simulink model "novamontagemrobo"  (R2018a)
settings: Solver=VariableStepAuto  StartTime=0.0  StopTime=59  FixedStep=0.4  MaxStep=0.4  RelTol=1e-3
model workspace: external: MATLAB File C:\Users\reigo\Downloads\robotica2\simulink_CERTO\simulink\novamontagemrobo_DataFile.m (data not in the file)
undefined symbols (not defined in the file or in its folder): smiData, X, Y, Z
libraries: sm_lib x57, nesl_utility x31
(part 3 of 3)

== matlab function novamontagemrobo/MATLAB Function3 ==
  data: parametro_robo input; T output; mass_robo input; valor_q_inv input; dq input; ddq input; inercia_robo input
function T = T(parametro_robo,mass_robo,valor_q_inv,dq,ddq,inercia_robo)

%T(E1,E2,Itarefa,L2,L3,L4,ddq1,ddq2,ddq3,ddq4,ddq5,ddq6,dq1,dq2,dq3,dq4,dq5,dq6,m2,m3,m4,m5,m6,m7,mtarefa,q1,q2,q3,q4,q5,q6,xf,yf,zf)


% parametro_robo=[L1,L2,L3,L4,E1,E2,xf,yf,zf];
% mass_robo=[mass1 mass2 mass3 mass4 mass5 mass6 mass7 masstarefa];
% inercia_robo=[inercia1 inercia2 inercia3 inercia4 inercia5 inercia6 inercia7 inerciatarefa];

coder.extrinsic('evalin');
T1 = evalin('caller','T1');
T2 = evalin('caller','T2');
T3 = evalin('caller','T3');
T4 = evalin('caller','T4');
T5 = evalin('caller','T5');
T6 = evalin('caller','T6');




L1=parametro_robo(1);
L2=parametro_robo(2);
L3=parametro_robo(3);
L4=parametro_robo(4);
E1=parametro_robo(5);
E2=parametro_robo(6);
xf=parametro_robo(7);
yf=parametro_robo(8);
zf=parametro_robo(9);


q1=valor_q_inv(1);
q2=valor_q_inv(2);
q3=valor_q_inv(3);
q4=valor_q_inv(4);
q5=valor_q_inv(5);
q6=valor_q_inv(6);


dq1=dq(1);
dq2=dq(2);
dq3=dq(3);
dq4=dq(4);
dq5=dq(5);
dq6=dq(6);



ddq1=ddq(1);
ddq2=ddq(2);
ddq3=ddq(3);
ddq4=ddq(4);
ddq5=ddq(5);
ddq6=ddq(6);

m1=mass_robo(1);
m2=mass_robo(2);
m3=mass_robo(3);
m4=mass_robo(4);
m5=mass_robo(5);
m6=mass_robo(6);
m7=mass_robo(7);
mtarefa=mass_robo(8);


Itarefa=inercia_robo(22:24,:);
Itarefaxx=Itarefa(1,1);
Itarefaxy=Itarefa(1,2);
Itarefaxz=Itarefa(1,3);
Itarefayx=Itarefa(2,1);
Itarefayy=Itarefa(2,2);
Itarefayz=Itarefa(2,3);
Itarefazx=Itarefa(3,1);
Itarefazy=Itarefa(3,2);
Itarefazz=Itarefa(3,3);


T1 = T1(E1,E2,Itarefaxx,Itarefaxy,Itarefayx,Itarefaxz,Itarefayy,Itarefazx,Itarefayz,Itarefazy,Itarefazz,L2,L3,L4,ddq1,ddq2,ddq3,ddq4,ddq5,ddq6,dq1,dq2,dq3,dq4,dq5,dq6,m2,m3,m4,m5,m6,m7,mtarefa,q1,q2,q3,q4,q5,q6,xf,yf,zf);
%T2 = T2(Itarefa,ddq1,ddq2,ddq3,ddq4,ddq5,ddq6,dq1,dq2,dq3,dq4,dq5,dq6,mtarefa,q1,q2,q3,q4,q5,q6);
T2 = T2(E1,E2,Itarefaxx,Itarefaxy,Itarefayx,Itarefaxz,Itarefayy,Itarefazx,Itarefayz,Itarefazy,Itarefazz,L2,L3,L4,ddq1,ddq2,ddq3,ddq4,ddq5,ddq6,dq1,dq2,dq3,dq4,dq5,dq6,m2,m3,m4,m5,m6,m7,mtarefa,q1,q2,q3,q4,q5,q6,xf,yf,zf);
T3 = T3(E1,E2,Itarefaxx,Itarefaxy,Itarefayx,Itarefaxz,Itarefayy,Itarefazx,Itarefayz,Itarefazy,Itarefazz,L2,L3,L4,ddq1,ddq2,ddq3,ddq4,ddq5,ddq6,dq1,dq2,dq3,dq4,dq5,dq6,m3,m4,m5,m6,m7,mtarefa,q1,q2,q3,q4,q5,q6,xf,yf,zf);
T4 = T4(E1,E2,Itarefaxx,Itarefaxy,Itarefayx,Itarefaxz,Itarefayy,Itarefazx,Itarefayz,Itarefazy,Itarefazz,L2,L3,L4,ddq1,ddq2,ddq3,ddq4,ddq5,ddq6,dq1,dq2,dq3,dq4,dq5,dq6,m4,m5,m6,m7,mtarefa,q1,q2,q3,q4,q5,q6,xf,yf,zf);
T5 = T5(E1,E2,Itarefaxx,Itarefaxy,Itarefayx,Itarefaxz,Itarefayy,Itarefazx,Itarefayz,Itarefazy,Itarefazz,L2,L3,L4,ddq1,ddq2,ddq3,ddq4,ddq5,ddq6,dq1,dq2,dq3,dq4,dq5,dq6,m5,m6,m7,mtarefa,q1,q2,q3,q4,q5,q6,xf,yf,zf);
T6 = T6(E1,E2,Itarefaxx,Itarefaxy,Itarefayx,Itarefaxz,Itarefayy,Itarefazx,Itarefayz,Itarefazy,Itarefazz,L2,L3,L4,ddq1,ddq2,ddq3,ddq4,ddq5,ddq6,dq1,dq2,dq3,dq4,dq5,dq6,m6,m7,mtarefa,q1,q2,q3,q4,q5,q6,xf,yf,zf);

T=zeros(6,1);
T = [T1; T2; T3; T4; T5; T6];

== matlab function novamontagemrobo/MATLAB Function4 ==
  data: matriz input; dq output; velocidades input
function dq = fcn(matriz,velocidades)

dq=matriz\velocidades';

== matlab function novamontagemrobo/MATLAB Function6 ==
  data: matriz input; ddq output; dq input; dmatriz input; aceleracao input
function ddq = acel_juntas(matriz,dq,dmatriz,aceleracao)


ddq=matriz\aceleracao'-matriz\dmatriz*dq;

== matlab function novamontagemrobo/djacob ==
  data: parametro_robo input; dJtot output; valor_q_inv input; dq input
function dJtot = djacob(parametro_robo,valor_q_inv,dq)
%#codegen

%    This function was generated by the Symbolic Math Toolbox version 8.1.
%    12-Jan-2021 01:39:36


L1=parametro_robo(1);
L2=parametro_robo(2);
L3=parametro_robo(3);
L4=parametro_robo(4);
E1=parametro_robo(5);
E2=parametro_robo(6);
xf=parametro_robo(7);
yf=parametro_robo(8);
zf=parametro_robo(9);


q1=valor_q_inv(1);
q2=valor_q_inv(2);
q3=valor_q_inv(3);
q4=valor_q_inv(4);
q5=valor_q_inv(5);
q6=valor_q_inv(6);


dq1=dq(1);
dq2=dq(2);
dq3=dq(3);
dq4=dq(4);
dq5=dq(5);
dq6=dq(6);




t2 = q2+q3;
t3 = sin(q1);
t4 = sin(q5);
t5 = cos(q1);
t6 = sin(q4);
t7 = t5.*t6;
t8 = sin(t2);
t9 = cos(q4);
t13 = t3.*t8.*t9;
t10 = t7-t13;
t11 = cos(t2);
t12 = cos(q5);
t14 = t4.*t10;
t15 = t3.*t11.*t12;
t16 = t14+t15;
t17 = sin(q6);
t18 = cos(q6);
t19 = t10.*t12;
t24 = t3.*t4.*t11;
t20 = t19-t24;
t21 = t5.*t9;
t22 = t3.*t6.*t8;
t23 = t21+t22;
t25 = L4+xf;
t26 = t3.*t4.*t8;
t42 = t3.*t9.*t11.*t12;
t27 = t26-t42;
t28 = cos(q2);
t29 = sin(q2);
t30 = t3.*t6;
t31 = t5.*t8.*t9;
t32 = t30+t31;
t33 = t3.*t9;
t102 = t5.*t6.*t8;
t34 = t33-t102;
t35 = t12.*t32;
t36 = t4.*t5.*t11;
t37 = t35+t36;
t38 = t3.*t8.*t12;
t39 = t3.*t4.*t9.*t11;
t40 = t38+t39;
t41 = t25.*t40;
t43 = t17.*t27;
t59 = t3.*t6.*t11.*t18;
t44 = t43-t59;
t45 = t44.*yf;
t46 = t18.*t27;
t47 = t3.*t6.*t11.*t17;
t48 = t46+t47;
t49 = t48.*zf;
t50 = t5.*t8.*t9.*t12;
t51 = t36+t50;
t52 = t5.*t8.*t12;
t53 = t4.*t5.*t9.*t11;
t54 = t52+t53;
t55 = L3.*t8;
t56 = L2.*t29;
t154 = E2.*t28;
t57 = t55+t56-t154;
t58 = t3.*t57;
t60 = t41+t45+t49+t58;
t61 = t4.*t5.*t8;
t63 = t5.*t9.*t11.*t12;
t62 = t61-t63;
t64 = t5.*t11.*t12;
t77 = t4.*t5.*t8.*t9;
t65 = t64-t77;
t66 = t25.*t65;
t67 = t17.*t51;
t68 = t5.*t6.*t8.*t18;
t69 = t67+t68;
t70 = t69.*yf;
t71 = t18.*t51;
t78 = t5.*t6.*t8.*t17;
t72 = t71-t78;
t73 = t72.*zf;
t74 = L3.*t11;
t75 = L2.*t28;
t76 = E2.*t29;
t79 = L3.*t5.*t11;
t80 = t66+t70+t73+t79;
t81 = t18.*t54.*zf;
t82 = t17.*t54.*yf;
t119 = t25.*t62;
t83 = t81+t82-t119;
t84 = t5.*t9.*t11.*t18;
t103 = t5.*t6.*t11.*t12.*t17;
t85 = t84-t103;
t86 = t85.*yf;
t87 = t5.*t9.*t11.*t17;
t88 = t5.*t6.*t11.*t12.*t18;
t89 = t87+t88;
t90 = t4.*t5.*t6.*t11.*t25;
t104 = t89.*zf;
t91 = t86+t90-t104;
t92 = dq4.*t91;
t93 = L3.*t3.*t8;
t94 = t41+t45+t49+t93;
t95 = t18.*t62;
t96 = t5.*t6.*t11.*t17;
t97 = t95+t96;
t98 = t97.*yf;
t99 = t17.*t62;
t145 = t5.*t6.*t11.*t18;
t100 = t99-t145;
t146 = t100.*zf;
t101 = t98-t146;
t105 = t10.*t18;
t106 = t12.*t17.*t23;
t107 = t105+t106;
t108 = t10.*t17;
t190 = t12.*t18.*t23;
t109 = t108-t190;
t110 = t109.*zf;
t111 = t4.*t23.*t25;
t112 = t110+t111-t107.*yf;
t113 = t18.*t34;
t114 = t17.*t34;
t115 = t20.*t25;
t116 = t16.*t18.*zf;
t117 = t16.*t17.*yf;
t118 = t115+t116+t117;
t120 = t12.*t25.*t34;
t121 = t4.*t18.*t34.*zf;
t122 = t4.*t17.*t34.*yf;
t123 = t120+t121+t122;
t124 = t4.*t32;
t125 = t64-t124;
t148 = t17.*t37;
t126 = t113-t148;
t127 = t126.*yf;
t128 = t18.*t37;
t129 = t114+t128;
t130 = t17.*t32;
t155 = t12.*t18.*t34;
t131 = t130-t155;
t132 = t131.*yf;
t133 = t18.*t32;
t134 = t12.*t17.*t34;
t135 = t133+t134;
t136 = t135.*zf;
t137 = t132+t136;
t138 = t17.*t23;
t139 = t18.*t20;
t140 = t138+t139;
t141 = t140.*yf;
t142 = t17.*t20;
t150 = t18.*t23;
t143 = t142-t150;
t144 = t141-t143.*zf;
t147 = t18.*t125.*yf;
t149 = E1+t74+t75+t76;
t151 = t25.*t54;
t152 = t100.*yf;
t153 = t97.*zf;
t156 = t74+t75+t76;
t157 = t3.*t8.*t9.*t12;
t158 = t24+t157;
t184 = t3.*t4.*t8.*t9;
t159 = t15-t184;
t160 = t25.*t159;
t161 = t17.*t158;
t162 = t3.*t6.*t8.*t18;
t163 = t161+t162;
t164 = t163.*yf;
t165 = t18.*t158;
t185 = t3.*t6.*t8.*t17;
t166 = t165-t185;
t167 = t166.*zf;
t168 = t5.*t57;
t169 = t151+t152+t153+t168;
t170 = L3.*t5.*t8;
t171 = t151+t152+t153+t170;
t172 = t18.*t40.*zf;
t173 = t17.*t40.*yf;
t197 = t25.*t27;
t174 = t172+t173-t197;
t175 = t3.*t9.*t11.*t18;
t191 = t3.*t6.*t11.*t12.*t17;
t176 = t175-t191;
t177 = t176.*yf;
t178 = t3.*t9.*t11.*t17;
t179 = t3.*t6.*t11.*t12.*t18;
t180 = t178+t179;
t181 = t3.*t4.*t6.*t11.*t25;
t192 = t180.*zf;
t182 = t177+t181-t192;
t183 = dq4.*t182;
t186 = L3.*t3.*t11;
t187 = t160+t164+t167+t186;
t188 = t48.*yf;
t212 = t44.*zf;
t189 = t188-t212;
t193 = t131.*zf;
t194 = t4.*t25.*t34;
t195 = t193+t194-t135.*yf;
t196 = t16.*t25;
t198 = t12.*t23.*t25;
t199 = t4.*t18.*t23.*zf;
t200 = t4.*t17.*t23.*yf;
t201 = t198+t199+t200;
t202 = t18.*t125.*zf;
t203 = t17.*t125.*yf;
t204 = t129.*yf;
t205 = t126.*zf;
t206 = t204+t205;
t207 = t109.*yf;
t208 = t107.*zf;
t209 = t207+t208;
t210 = t16.*t18.*yf;
t211 = t210-t16.*t17.*zf;
t213 = t11.*t12;
t232 = t4.*t8.*t9;
t214 = t213-t232;
t215 = t4.*t8;
t217 = t9.*t11.*t12;
t216 = t215-t217;
t218 = t17.*t216;
t244 = t6.*t11.*t18;
t219 = t218-t244;
t220 = t219.*yf;
t221 = t18.*t216;
t222 = t6.*t11.*t17;
t223 = t221+t222;
t224 = t223.*zf;
t225 = t8.*t12;
t226 = t4.*t9.*t11;
t227 = t225+t226;
t228 = t25.*t227;
t229 = t4.*t11;
t230 = t8.*t9.*t12;
t231 = t229+t230;
t233 = t18.*t214.*zf;
t234 = t17.*t214.*yf;
t255 = t25.*t231;
t235 = t233+t234-t255;
t236 = t8.*t9.*t18;
t253 = t6.*t8.*t12.*t17;
t237 = t236-t253;
t238 = t237.*yf;
t239 = t8.*t9.*t17;
t240 = t6.*t8.*t12.*t18;
t241 = t239+t240;
t242 = t4.*t6.*t8.*t25;
t254 = t241.*zf;
t243 = t238+t242-t254;
t245 = t55+t220+t224+t228;
t246 = dq3.*t245;
t247 = t18.*t231;
t270 = t6.*t8.*t17;
t248 = t247-t270;
t249 = t17.*t231;
t250 = t6.*t8.*t18;
t251 = t249+t250;
t271 = t248.*yf;
t272 = t251.*zf;
t252 = t271-t272;
t256 = t6.*t11.*t12.*t25;
t257 = t4.*t6.*t11.*t18.*zf;
t258 = t4.*t6.*t11.*t17.*yf;
t259 = t256+t257+t258;
t260 = t9.*t11.*t17;
t261 = t6.*t11.*t12.*t18;
t262 = t260+t261;
t263 = t262.*yf;
t264 = t9.*t11.*t18;
t265 = t264-t6.*t11.*t12.*t17;
t266 = t265.*zf;
t267 = t263+t266;
t268 = t18.*t227.*yf;
t269 = t268-t17.*t227.*zf;
dJtot = reshape([dq2.*t60+dq3.*t94-dq4.*t112-dq5.*t118+dq6.*t144+dq1.*(t127-t5.*t149-t129.*zf+t25.*(t124-t5.*t11.*t12)),-dq2.*t169-dq3.*t171-dq4.*t195+dq6.*t206+dq5.*(t202+t203-t25.*t37)-dq1.*(t196+t3.*t149-t143.*yf-t140.*zf),0.0,0.0,0.0,0.0,t92+dq1.*t60-dq3.*t80-dq5.*t83-dq6.*t101-dq2.*(t66+t70+t73+t5.*t156),t183-dq1.*t169-dq5.*t174-dq3.*t187-dq6.*t189-dq2.*(t160+t164+t167+t3.*t156),t246-dq5.*t235-dq4.*t243-dq6.*t252+dq2.*(t55+t56-t154+t220+t224+t228),-dq1.*t5,-dq1.*t3,0.0,t92-dq2.*t80-dq3.*t80-dq5.*t83+dq1.*t94-dq6.*t101,t183-dq1.*t171-dq5.*t174-dq2.*t187-dq3.*t187-dq6.*t189,t246-dq5.*t235+dq2.*t245-dq4.*t243-dq6.*t252,-dq1.*t5,-dq1.*t3,0.0,dq2.*t91+dq3.*t91-dq1.*t112-dq5.*t123-dq6.*t137+dq4.*(yf.*(t113-t12.*t17.*t32)-zf.*(t114+t12.*t18.*t32)+t4.*t25.*t32),dq2.*t182+dq3.*t182-dq1.*t195+dq5.*t201+dq6.*t209-dq4.*(yf.*(t150-t10.*t12.*t17)-zf.*(t138+t10.*t12.*t18)+t4.*t10.*t25),dq4.*(-yf.*(t244+t9.*t11.*t12.*t17)+zf.*(t222-t9.*t11.*t12.*t18)+t4.*t9.*t11.*t25)-dq2.*t243-dq3.*t243+dq5.*t259-dq6.*t267,-dq1.*t3.*t11-dq2.*t5.*t8-dq3.*t5.*t8,-dq2.*t3.*t8-dq3.*t3.*t8+dq1.*t5.*t11,-dq2.*t11-dq3.*t11,-dq2.*t83-dq3.*t83-dq1.*t118-dq4.*t123+dq6.*(t147-t17.*t125.*zf)-dq5.*(t25.*t125+t17.*t37.*yf+t18.*t37.*zf),-dq2.*t174-dq3.*t174+dq4.*t201+dq6.*t211+dq1.*(t202+t203-t25.*t37)+dq5.*(-t196+t17.*t20.*yf+t18.*t20.*zf),dq5.*(t228+t17.*t216.*yf+t18.*t216.*zf)-dq2.*t235-dq3.*t235+dq4.*t259-dq6.*t269,-dq1.*t23+dq4.*t32+dq2.*t5.*t6.*t11+dq3.*t5.*t6.*t11,-dq4.*t10-dq1.*t34+dq2.*t3.*t6.*t11+dq3.*t3.*t6.*t11,-dq2.*t6.*t8-dq3.*t6.*t8+dq4.*t9.*t11,-dq2.*t101-dq3.*t101-dq4.*t137+dq1.*t144+dq5.*(t147-t17.*zf.*(t64-t124))+dq6.*(t127-t129.*zf),-dq2.*t189-dq3.*t189+dq1.*t206+dq4.*t209+dq5.*t211+dq6.*(t143.*yf+t140.*zf),dq6.*(t220+t224)-dq2.*t252-dq3.*t252-dq4.*t267-dq5.*t269,-dq1.*t16-dq5.*t37-dq2.*t54-dq3.*t54-dq4.*t4.*t34,dq5.*t20-dq2.*t40-dq3.*t40+dq1.*(t64-t124)+dq4.*t4.*t23,-dq2.*t214-dq3.*t214+dq5.*t216+dq4.*t4.*t6.*t11],[6,6]);

== matlab function novamontagemrobo/jacob ==
  data: parametro_robo input; Jtot output; valor_q_inv input
function Jtot = jacob(parametro_robo,valor_q_inv)
%#codegen

%    This function was generated by the Symbolic Math Toolbox version 8.1.
%    12-Jan-2021 01:39:21


L1=parametro_robo(1);
L2=parametro_robo(2);
L3=parametro_robo(3);
L4=parametro_robo(4);
E1=parametro_robo(5);
E2=parametro_robo(6);
xf=parametro_robo(7);
yf=parametro_robo(8);
zf=parametro_robo(9);


q1=valor_q_inv(1);
q2=valor_q_inv(2);
q3=valor_q_inv(3);
q4=valor_q_inv(4);
q5=valor_q_inv(5);
q6=valor_q_inv(6);



t2 = q2+q3;
t3 = sin(q1);
t4 = cos(t2);
t5 = cos(q1);
t6 = cos(q4);
t7 = sin(t2);
t8 = sin(q4);
t9 = cos(q5);
t10 = t5.*t8;
t18 = t3.*t6.*t7;
t11 = t10-t18;
t12 = sin(q5);
t13 = sin(q6);
t14 = t5.*t6;
t15 = t3.*t7.*t8;
t16 = t14+t15;
t17 = cos(q6);
t19 = t9.*t11;
t70 = t3.*t4.*t12;
t20 = t19-t70;
t21 = L4+xf;
t22 = t5.*t7.*t12;
t29 = t4.*t5.*t6.*t9;
t23 = t22-t29;
t24 = cos(q2);
t25 = sin(q2);
t26 = t5.*t7.*t9;
t27 = t4.*t5.*t6.*t12;
t28 = t26+t27;
t30 = t13.*t23;
t31 = t30-t4.*t5.*t8.*t17;
t32 = t17.*t23;
t33 = t4.*t5.*t8.*t13;
t34 = t32+t33;
t35 = t3.*t8;
t36 = t5.*t6.*t7;
t37 = t35+t36;
t38 = t3.*t6;
t40 = t5.*t7.*t8;
t39 = t38-t40;
t41 = t12.*t37;
t46 = t4.*t5.*t9;
t42 = t41-t46;
t43 = t9.*t37;
t44 = t4.*t5.*t12;
t45 = t43+t44;
t47 = L3.*t4;
t48 = L2.*t24;
t49 = E2.*t25;
t50 = E1+t47+t48+t49;
t51 = t17.*t39;
t52 = t51-t13.*t45;
t53 = t13.*t39;
t54 = t17.*t45;
t55 = t53+t54;
t56 = L3.*t7;
t57 = L2.*t25;
t58 = t56+t57-E2.*t24;
t59 = t3.*t7.*t12;
t64 = t3.*t4.*t6.*t9;
t60 = t59-t64;
t61 = t3.*t7.*t9;
t62 = t3.*t4.*t6.*t12;
t63 = t61+t62;
t65 = t13.*t60;
t66 = t65-t3.*t4.*t8.*t17;
t67 = t17.*t60;
t68 = t3.*t4.*t8.*t13;
t69 = t67+t68;
t71 = t11.*t12;
t72 = t3.*t4.*t9;
t73 = t71+t72;
t74 = t13.*t16;
t75 = t17.*t20;
t76 = t74+t75;
t77 = t13.*t20;
t78 = t4.*t12;
t79 = t6.*t7.*t9;
t80 = t78+t79;
t81 = t13.*t80;
t82 = t7.*t8.*t17;
t83 = t81+t82;
t84 = t17.*t80;
t85 = t84-t7.*t8.*t13;
t86 = t4.*t9;
t87 = t86-t6.*t7.*t12;
t88 = t7.*t9;
t89 = t4.*t6.*t12;
t90 = t88+t89;
t91 = t7.*t12;
t93 = t4.*t6.*t9;
t92 = t91-t93;
Jtot = reshape([-t3.*t50-t21.*t73+t76.*zf+yf.*(t77-t16.*t17),t5.*t50-t21.*t42-t52.*yf+t55.*zf,0.0,0.0,0.0,1.0,-t21.*t28-t5.*t58-t31.*yf-t34.*zf,-t3.*t58-t21.*t63-t66.*yf-t69.*zf,-t47-t48-t49-t21.*t87-t83.*yf-t85.*zf,-t3,t5,0.0,-t21.*t28-t31.*yf-t34.*zf-L3.*t5.*t7,-t21.*t63-t66.*yf-t69.*zf-L3.*t3.*t7,-t47-t21.*t87-t83.*yf-t85.*zf,-t3,t5,0.0,yf.*(t17.*t37+t9.*t13.*t39)-zf.*(t13.*t37-t9.*t17.*t39)-t12.*t21.*t39,-yf.*(t11.*t17+t9.*t13.*t16)+zf.*(t11.*t13-t9.*t16.*t17)+t12.*t16.*t21,yf.*(t4.*t6.*t17-t4.*t8.*t9.*t13)-zf.*(t4.*t6.*t13+t4.*t8.*t9.*t17)+t4.*t8.*t12.*t21,t4.*t5,t3.*t4,-t7,-t21.*t45-t13.*t42.*yf-t17.*t42.*zf,t20.*t21+t13.*t73.*yf+t17.*t73.*zf,t21.*t92-t13.*t90.*yf-t17.*t90.*zf,-t38+t40,t16,t4.*t8,t55.*yf+t52.*zf,-t76.*yf+zf.*(t77-t16.*t17),-yf.*(t17.*t92+t4.*t8.*t13)+zf.*(t13.*t92-t4.*t8.*t17),-t41+t46,t73,-t88-t89],[6,6]);

== matlab function novamontagemrobo/MATLAB Function7 ==
  data: parametro_robo output; config_tarefa output; massa_robo output; inercia_robo output
function [parametro_robo,config_tarefa,massa_robo,inercia_robo] = condicao_inicial
L1=0.590; L2=1.350; L3=1.600;L4=0.215;
E1=0.750; E2=-0.041;
xf=0.22485;yf=0;zf=0;


mass1=207.61613;
mass2=346.81729;
mass3=366.65763;
mass4=243.34094;
mass5=10.76884;
mass6=27.61521;
mass7=3.40236; %flange+ferramenta
masstarefa=8.90300;
%masstarefa=0;



inercia1=[6.45927 0.00073 -0.42267; 0.00073 8.55120 0.00155; -0.42267 0.00155 13.15421];

%

inercia2=[11.08697 3.39167 5.38787; 3.39167 37.87049 0.88684; 5.38787 0.88684 35.38487];  % Kg*m^2 
inercia3=[6.70839 -7.30351 -0.12339; -7.30351 78.03742 0.03995; -0.12339 0.03995 78.85343];
inercia4=[2.40106 1.64045 -1.15010; 1.64045 48.35669 -0.11971; -1.15010 -0.11971 47.88720];
inercia5=[0.02668 0.00251 0.00000; 0.00251 0.11156 0.00000; 0.00000 0.00000 0.10998];
inercia6=[0.26923 -0.04332 -0.00012; -0.04332 0.22283 -0.00011; -0.00012 -0.00011 0.37601];
inercia7=[0.05118 -0.0005 -0.00002; -0.00005 0.01547 0.00003; -0.00002 0.00003 0.06098]; %flange+ferramenta
inerciatarefa=[0.22649 -0.00006 -0.00005;-0.00006 0.17109 -0.00013;-0.00005 -0.00013 0.23614];

%inerciatarefa=zeros(3,3);








%ligar desligar mtarefa e inerciatarefa daqui. alterar função para receber
%tempo


parametro_robo=[L1,L2,L3,L4,E1,E2,xf,yf,zf];
massa_robo=[mass1 mass2 mass3 mass4 mass5 mass6 mass7 masstarefa];
inercia_robo=[inercia1; inercia2 ;inercia3 ;inercia4 ;inercia5 ;inercia6 ;inercia7 ;inerciatarefa];
%inercia_robo=inerciatarefa;
xC = 0; yC = 0; zC = 0; qxC = 0; qyC = 0; qzC = 0; 
alt_min_eixo2=0.585;
config_tarefa=[xC,yC,zC,qxC,qyC,qzC,alt_min_eixo2];

end

== matlab function novamontagemrobo/MATLAB Function9 ==
  data: parametro_robo input; G output; mass_robo input; valor_q_inv input
function G = G(parametro_robo,mass_robo,valor_q_inv)

coder.extrinsic('evalin');
G1 = evalin('caller','G1'); 
G2 = evalin('caller','G2');
G3 = evalin('caller','G3');
G4 = evalin('caller','G4');
G5 = evalin('caller','G5');
G6 = evalin('caller','G6');




L1=parametro_robo(1);
L2=parametro_robo(2);
L3=parametro_robo(3);
L4=parametro_robo(4);
E1=parametro_robo(5);
E2=parametro_robo(6);
xf=parametro_robo(7);
yf=parametro_robo(8);
zf=parametro_robo(9);


q1=valor_q_inv(1);
q2=valor_q_inv(2);
q3=valor_q_inv(3);
q4=valor_q_inv(4);
q5=valor_q_inv(5);
q6=valor_q_inv(6);



m1=mass_robo(1);
m2=mass_robo(2);
m3=mass_robo(3);
m4=mass_robo(4);
m5=mass_robo(5);
m6=mass_robo(6);
m7=mass_robo(7);
mtarefa=mass_robo(8);




G1 = G1();
G2 = G2(E2,L2,L3,L4,m2,m3,m4,m5,m6,m7,mtarefa,q2,q3,q4,q5,q6,xf,yf,zf);
G3 = G3(E2,L3,L4,m3,m4,m5,m6,m7,mtarefa,q2,q3,q4,q5,q6,xf,yf,zf);
G4 = G4(L4,m4,m5,m6,m7,mtarefa,q2,q3,q4,q5,q6,xf,yf,zf);
G5 = G5(L4,m5,m6,m7,mtarefa,q2,q3,q4,q5,q6,xf,yf,zf);
G6 = G6(m6,m7,mtarefa,q2,q3,q4,q5,q6,yf,zf);

G=zeros(6,1);
G = [G1; G2; G3; G4; G5; G6];

== matlab function novamontagemrobo/MATLAB Function10 ==
  data: T input; H output; M input; ddq input; G input
function H = H(T, M ,ddq, G)

H = T-M*ddqm-G;

== matlab function novamontagemrobo/MATLAB Function11 ==
  data: T input; H output; M input; ddq input; G input
function H = H(T, M ,ddq, G)

H = T-M*ddq-G;

== matlab function novamontagemrobo/MATLAB Function12 ==
  data: parametro_robo input; T output; mass_robo input; qm input; dqm input; ddqm input; inercia_robo input
function T = T(parametro_robo,mass_robo,qm,dqm,ddqm,inercia_robo)

%T(E1,E2,Itarefa,L2,L3,L4,ddq1,ddq2,ddq3,ddq4,ddq5,ddq6,dq1,dq2,dq3,dq4,dq5,dq6,m2,m3,m4,m5,m6,m7,mtarefa,q1,q2,q3,q4,q5,q6,xf,yf,zf)


% parametro_robo=[L1,L2,L3,L4,E1,E2,xf,yf,zf];
% mass_robo=[mass1 mass2 mass3 mass4 mass5 mass6 mass7 masstarefa];
% inercia_robo=[inercia1 inercia2 inercia3 inercia4 inercia5 inercia6 inercia7 inerciatarefa];


coder.extrinsic('evalin');
T1 = evalin('caller','T1');
T2 = evalin('caller','T2');
T3 = evalin('caller','T3');
T4 = evalin('caller','T4');
T5 = evalin('caller','T5');
T6 = evalin('caller','T6');



L1=parametro_robo(1);
L2=parametro_robo(2);
L3=parametro_robo(3);
L4=parametro_robo(4);
E1=parametro_robo(5);
E2=parametro_robo(6);
xf=parametro_robo(7);
yf=parametro_robo(8);
zf=parametro_robo(9);


q1=qm(1);
q2=qm(2);
q3=qm(3);
q4=qm(4);
q5=qm(5);
q6=qm(6);


dq1=dqm(1);
dq2=dqm(2);
dq3=dqm(3);
dq4=dqm(4);
dq5=dqm(5);
dq6=dqm(6);



ddq1=ddqm(1);
ddq2=ddqm(2);
ddq3=ddqm(3);
ddq4=ddqm(4);
ddq5=ddqm(5);
ddq6=ddqm(6);

m1=mass_robo(1);
m2=mass_robo(2);
m3=mass_robo(3);
m4=mass_robo(4);
m5=mass_robo(5);
m6=mass_robo(6);
m7=mass_robo(7);
mtarefa=mass_robo(8);


Itarefa=inercia_robo(22:24,:);
Itarefaxx=Itarefa(1,1);
Itarefaxy=Itarefa(1,2);
Itarefaxz=Itarefa(1,3);
Itarefayx=Itarefa(2,1);
Itarefayy=Itarefa(2,2);
Itarefayz=Itarefa(2,3);
Itarefazx=Itarefa(3,1);
Itarefazy=Itarefa(3,2);
Itarefazz=Itarefa(3,3);


T1 = T1(E1,E2,Itarefaxx,Itarefaxy,Itarefayx,Itarefaxz,Itarefayy,Itarefazx,Itarefayz,Itarefazy,Itarefazz,L2,L3,L4,ddq1,ddq2,ddq3,ddq4,ddq5,ddq6,dq1,dq2,dq3,dq4,dq5,dq6,m2,m3,m4,m5,m6,m7,mtarefa,q1,q2,q3,q4,q5,q6,xf,yf,zf);
%T2 = T2(Itarefa,ddq1,ddq2,ddq3,ddq4,ddq5,ddq6,dq1,dq2,dq3,dq4,dq5,dq6,mtarefa,q1,q2,q3,q4,q5,q6);
T2 = T2(E1,E2,Itarefaxx,Itarefaxy,Itarefayx,Itarefaxz,Itarefayy,Itarefazx,Itarefayz,Itarefazy,Itarefazz,L2,L3,L4,ddq1,ddq2,ddq3,ddq4,ddq5,ddq6,dq1,dq2,dq3,dq4,dq5,dq6,m2,m3,m4,m5,m6,m7,mtarefa,q1,q2,q3,q4,q5,q6,xf,yf,zf);
T3 = T3(E1,E2,Itarefaxx,Itarefaxy,Itarefayx,Itarefaxz,Itarefayy,Itarefazx,Itarefayz,Itarefazy,Itarefazz,L2,L3,L4,ddq1,ddq2,ddq3,ddq4,ddq5,ddq6,dq1,dq2,dq3,dq4,dq5,dq6,m3,m4,m5,m6,m7,mtarefa,q1,q2,q3,q4,q5,q6,xf,yf,zf);
T4 = T4(E1,E2,Itarefaxx,Itarefaxy,Itarefayx,Itarefaxz,Itarefayy,Itarefazx,Itarefayz,Itarefazy,Itarefazz,L2,L3,L4,ddq1,ddq2,ddq3,ddq4,ddq5,ddq6,dq1,dq2,dq3,dq4,dq5,dq6,m4,m5,m6,m7,mtarefa,q1,q2,q3,q4,q5,q6,xf,yf,zf);
T5 = T5(E1,E2,Itarefaxx,Itarefaxy,Itarefayx,Itarefaxz,Itarefayy,Itarefazx,Itarefayz,Itarefazy,Itarefazz,L2,L3,L4,ddq1,ddq2,ddq3,ddq4,ddq5,ddq6,dq1,dq2,dq3,dq4,dq5,dq6,m5,m6,m7,mtarefa,q1,q2,q3,q4,q5,q6,xf,yf,zf);
T6 = T6(E1,E2,Itarefaxx,Itarefaxy,Itarefayx,Itarefaxz,Itarefayy,Itarefazx,Itarefayz,Itarefazy,Itarefazz,L2,L3,L4,ddq1,ddq2,ddq3,ddq4,ddq5,ddq6,dq1,dq2,dq3,dq4,dq5,dq6,m6,m7,mtarefa,q1,q2,q3,q4,q5,q6,xf,yf,zf);

T=zeros(6,1);
T = [T1; T2; T3; T4; T5; T6];

== matlab function novamontagemrobo/MATLAB Function13 ==
  data: parametro_robo input; M output; mass_robo input; qm input; inercia_robo input
function M = M(parametro_robo,mass_robo,qm,inercia_robo)

%T(E1,E2,Itarefa,L2,L3,L4,ddq1,ddq2,ddq3,ddq4,ddq5,ddq6,dq1,dq2,dq3,dq4,dq5,dq6,m2,m3,m4,m5,m6,m7,mtarefa,q1,q2,q3,q4,q5,q6,xf,yf,zf)


% parametro_robo=[L1,L2,L3,L4,E1,E2,xf,yf,zf];
% mass_robo=[mass1 mass2 mass3 mass4 mass5 mass6 mass7 masstarefa];
% inercia_robo=[inercia1 inercia2 inercia3 inercia4 inercia5 inercia6 inercia7 inerciatarefa];

coder.extrinsic('evalin');
M1 = evalin('caller','M1');
M2 = evalin('caller','M2');
M3 = evalin('caller','M3');
M4 = evalin('caller','M4');
M5 = evalin('caller','M5');
M6 = evalin('caller','M6');

L1=parametro_robo(1);
L2=parametro_robo(2);
L3=parametro_robo(3);
L4=parametro_robo(4);
E1=parametro_robo(5);
E2=parametro_robo(6);
xf=parametro_robo(7);
yf=parametro_robo(8);
zf=parametro_robo(9);


q1=qm(1);
q2=qm(2);
q3=qm(3);
q4=qm(4);
q5=qm(5);
q6=qm(6);



m1=mass_robo(1);
m2=mass_robo(2);
m3=mass_robo(3);
m4=mass_robo(4);
m5=mass_robo(5);
m6=mass_robo(6);
m7=mass_robo(7);
mtarefa=mass_robo(8);


Itarefa=inercia_robo(22:24,:);
Itarefaxx=Itarefa(1,1);
Itarefaxy=Itarefa(1,2);
Itarefaxz=Itarefa(1,3);
Itarefayx=Itarefa(2,1);
Itarefayy=Itarefa(2,2);
Itarefayz=Itarefa(2,3);
Itarefazx=Itarefa(3,1);
Itarefazy=Itarefa(3,2);
Itarefazz=Itarefa(3,3);


M1 = M1(E1,E2,Itarefaxx,Itarefaxy,Itarefayx,Itarefaxz,Itarefayy,Itarefazx,Itarefayz,Itarefazy,Itarefazz,L2,L3,L4,m2,m3,m4,m5,m6,m7,mtarefa,q1,q2,q3,q4,q5,q6,xf,yf,zf);
M2 = M2(E1,E2,Itarefaxx,Itarefaxy,Itarefayx,Itarefaxz,Itarefayy,Itarefazx,Itarefayz,Itarefazy,Itarefazz,L2,L3,L4,m2,m3,m4,m5,m6,m7,mtarefa,q1,q2,q3,q4,q5,q6,xf,yf,zf);
M3 = M3(E1,E2,Itarefaxx,Itarefaxy,Itarefayx,Itarefaxz,Itarefayy,Itarefazx,Itarefayz,Itarefazy,Itarefazz,L2,L3,L4,m3,m4,m5,m6,m7,mtarefa,q1,q2,q3,q4,q5,q6,xf,yf,zf);
M4 = M4(E1,E2,Itarefaxx,Itarefaxy,Itarefayx,Itarefaxz,Itarefayy,Itarefazx,Itarefayz,Itarefazy,Itarefazz,L2,L3,L4,m4,m5,m6,m7,mtarefa,q1,q2,q3,q4,q5,q6,xf,yf,zf);
M5 = M5(E1,E2,Itarefaxx,Itarefaxy,Itarefayx,Itarefaxz,Itarefayy,Itarefazx,Itarefayz,Itarefazy,Itarefazz,L2,L3,L4,m5,m6,m7,mtarefa,q1,q2,q3,q4,q5,q6,xf,yf,zf);
M6 = M6(E1,E2,Itarefaxx,Itarefaxy,Itarefayx,Itarefaxz,Itarefayy,Itarefazx,Itarefayz,Itarefazy,Itarefazz,L2,L3,L4,m6,m7,mtarefa,q1,q2,q3,q4,q5,q6,xf,yf,zf);

M=zeros(6,6);
M = [M1; M2; M3; M4; M5; M6];

== matlab function novamontagemrobo/MATLAB Function14 ==
  data: parametro_robo input; G output; mass_robo input; qm input
function G = G(parametro_robo,mass_robo,qm)

coder.extrinsic('evalin');
G1 = evalin('caller','G1'); 
G2 = evalin('caller','G2');
G3 = evalin('caller','G3');
G4 = evalin('caller','G4');
G5 = evalin('caller','G5');
G6 = evalin('caller','G6');


L1=parametro_robo(1);
L2=parametro_robo(2);
L3=parametro_robo(3);
L4=parametro_robo(4);
E1=parametro_robo(5);
E2=parametro_robo(6);
xf=parametro_robo(7);
yf=parametro_robo(8);
zf=parametro_robo(9);


q1=qm(1);
q2=qm(2);
q3=qm(3);
q4=qm(4);
q5=qm(5);
q6=qm(6);



m1=mass_robo(1);
m2=mass_robo(2);
m3=mass_robo(3);
m4=mass_robo(4);
m5=mass_robo(5);
m6=mass_robo(6);
m7=mass_robo(7);
mtarefa=mass_robo(8);




G1 = G1();
G2 = G2(E2,L2,L3,L4,m2,m3,m4,m5,m6,m7,mtarefa,q2,q3,q4,q5,q6,xf,yf,zf);
G3 = G3(E2,L3,L4,m3,m4,m5,m6,m7,mtarefa,q2,q3,q4,q5,q6,xf,yf,zf);
G4 = G4(L4,m4,m5,m6,m7,mtarefa,q2,q3,q4,q5,q6,xf,yf,zf);
G5 = G5(L4,m5,m6,m7,mtarefa,q2,q3,q4,q5,q6,xf,yf,zf);
G6 = G6(m6,m7,mtarefa,q2,q3,q4,q5,q6,yf,zf);

G=zeros(6,1);
G = [G1; G2; G3; G4; G5; G6];

== matlab function novamontagemrobo/MATLAB Function15 ==
  data: posX output; posY output; parametro_robo input; valor_q_inv input; posZ output; tarefa input; qx output; qy output; qz output; caixa input
function [posX,posY,posZ,qx,qy,qz] = pos_caixa1(parametro_robo,valor_q_inv,tarefa,caixa)
coder.extrinsic('evalin')
qx=(pi/2);
qy=(pi/2)+pi/2;
qz=0;
xf=parametro_robo(7);
posX=0;
posY=2.5-xf;
posZ=0.90764;

if caixa>1
    posX=0.19985;
    posY=-2.04985+xf;
    posZ= 0.24564;
    qy=0;
end

if caixa==1
qx=tarefa(4)+(pi/2);
qy=tarefa(6)+(pi/2);
qz=-tarefa(5);
L1=parametro_robo(1);L2=parametro_robo(2); L3=parametro_robo(3);L4=parametro_robo(4);
E1=parametro_robo(5);E2=parametro_robo(6);yf=parametro_robo(8);
zf=parametro_robo(9);


q1=valor_q_inv(1);q2=valor_q_inv(2);q3=valor_q_inv(3);q4=valor_q_inv(4);
q5=valor_q_inv(5);q6=valor_q_inv(6);


 R1_0 = [cos(q1) -sin(q1) 0 0; sin(q1) cos(q1) 0 0; 0 0 1 0; 0 0 0 1];
 D1_0 = [1 0 0 E1; 0 1 0 0; 0 0 1 L1; 0 0 0 1];
 T1_0 = R1_0*D1_0;
 R2_1 = [cos(q2) 0 sin(q2) 0; 0 1 0 0; -sin(q2) 0 cos(q2) 0; 0 0 0 1];
 D2_1 = [1 0 0 L2; 0 1 0 0; 0 0 1 0; 0 0 0 1];
 T2_1 = R2_1*D2_1;
 T2_0 = T1_0*T2_1;
 R3_2 = [cos(q3) 0 sin(q3) 0; 0 1 0 0; -sin(q3) 0 cos(q3) 0; 0 0 0 1];
 D3_2 = [1 0 0 L3; 0 1 0 0; 0 0 1 E2; 0 0 0 1];
 T3_2 = R3_2*D3_2;
 T3_0 = T2_0*T3_2;
 R4_3 = [1 0 0 0; 0 cos(q4) -sin(q4) 0; 0 sin(q4) cos(q4) 0; 0 0 0 1];
 T4_3 = R4_3;
 T4_0 =T3_0*T4_3;
 R5_4 = [cos(q5) 0 sin(q5) 0; 0 1 0 0; -sin(q5) 0 cos(q5) 0; 0 0 0 1];
 T5_4 = R5_4;
 T5_0 = T4_0*T5_4;                               
 R6_5 = [1 0 0 0; 0 cos(q6) -sin(q6) 0; 0 sin(q6) cos(q6) 0; 0 0 0 1];
 T6_5 = R6_5;
 T6_0 = T5_0*T6_5; 
 D7_6 = [1 0 0 L4; 0 1 0 yf; 0 0 1 zf; 0 0 0 1];
 T7_6 = D7_6;
 T7_0=T6_0*T7_6;
 pos=T7_0(1:3,4);
posX=pos(1);
posY=pos(2);
posZ=pos(3);
end
end

== matlab function novamontagemrobo/MATLAB Function16 ==
  data: posX output; posY output; parametro_robo input; valor_q_inv input; posZ output; tarefa input; qx output; qy output; qz output; caixa input
function [posX,posY,posZ,qx,qy,qz] = pos_caixa3(parametro_robo,valor_q_inv,tarefa,caixa)
coder.extrinsic('evalin')
qx=(pi/2);
qy=(pi/2)+pi/2;
qz=0;
xf=parametro_robo(7);
posX=0;
posY=3.1-xf;
posZ=0.9076;

if caixa>=2 && caixa<4
    posX=0;
    posY=2.8-xf;
    posZ=0.90764;
end

if caixa==4
    posX=0;
    posY=2.5-xf;
    posZ=0.90764;
end

if caixa>5
    posX=0.19985;
    posY=-2.04985+xf;
    posZ= 0.58564;
    qy=0;
end

if caixa==5
qx=tarefa(4)+(pi/2);
qy=tarefa(6)+(pi/2);
qz=-tarefa(5);
L1=parametro_robo(1);L2=parametro_robo(2); L3=parametro_robo(3);L4=parametro_robo(4);
E1=parametro_robo(5);E2=parametro_robo(6);yf=parametro_robo(8);
zf=parametro_robo(9);


q1=valor_q_inv(1);q2=valor_q_inv(2);q3=valor_q_inv(3);q4=valor_q_inv(4);
q5=valor_q_inv(5);q6=valor_q_inv(6);


 R1_0 = [cos(q1) -sin(q1) 0 0; sin(q1) cos(q1) 0 0; 0 0 1 0; 0 0 0 1];
 D1_0 = [1 0 0 E1; 0 1 0 0; 0 0 1 L1; 0 0 0 1];
 T1_0 = R1_0*D1_0;
 R2_1 = [cos(q2) 0 sin(q2) 0; 0 1 0 0; -sin(q2) 0 cos(q2) 0; 0 0 0 1];
 D2_1 = [1 0 0 L2; 0 1 0 0; 0 0 1 0; 0 0 0 1];
 T2_1 = R2_1*D2_1;
 T2_0 = T1_0*T2_1;
 R3_2 = [cos(q3) 0 sin(q3) 0; 0 1 0 0; -sin(q3) 0 cos(q3) 0; 0 0 0 1];
 D3_2 = [1 0 0 L3; 0 1 0 0; 0 0 1 E2; 0 0 0 1];
 T3_2 = R3_2*D3_2;
 T3_0 = T2_0*T3_2;
 R4_3 = [1 0 0 0; 0 cos(q4) -sin(q4) 0; 0 sin(q4) cos(q4) 0; 0 0 0 1];
 T4_3 = R4_3;
 T4_0 =T3_0*T4_3;
 R5_4 = [cos(q5) 0 sin(q5) 0; 0 1 0 0; -sin(q5) 0 cos(q5) 0; 0 0 0 1];
 T5_4 = R5_4;
 T5_0 = T4_0*T5_4;                               
 R6_5 = [1 0 0 0; 0 cos(q6) -sin(q6) 0; 0 sin(q6) cos(q6) 0; 0 0 0 1];
 T6_5 = R6_5;
 T6_0 = T5_0*T6_5; 
 D7_6 = [1 0 0 L4; 0 1 0 yf; 0 0 1 zf; 0 0 0 1];
 T7_6 = D7_6;
 T7_0=T6_0*T7_6;
 pos=T7_0(1:3,4);
posX=pos(1);
posY=pos(2);
posZ=pos(3);
end
end

== matlab function novamontagemrobo/MATLAB Function17 ==
  data: posX output; posY output; parametro_robo input; valor_q_inv input; posZ output; tarefa input; qx output; qy output; qz output; caixa input
function [posX,posY,posZ,qx,qy,qz] = pos_caixa4(parametro_robo,valor_q_inv,tarefa,caixa)
coder.extrinsic('evalin')
qx=(pi/2);
qy=(pi/2)+pi/2;
qz=0;
xf=parametro_robo(7);
posX=0;
posY=3.4-xf;
posZ=0.9076;

if caixa>=2 && caixa<4
    posX=0;
    posY=3.1-xf;
    posZ=0.90764;
end

if caixa>=4 && caixa <6
    posX=0;
    posY=2.8-xf;
    posZ=0.90764;
end

if caixa==6
    posX=0;
    posY=2.5-xf;
    posZ=0.90764;
end


if caixa>7
    posX=0.80015;
    posY=-2.04985+xf;
    posZ= 0.58564;
    qy=0;
end

if caixa==7
qx=tarefa(4)+(pi/2);
qy=tarefa(6)+(pi/2);
qz=-tarefa(5);
L1=parametro_robo(1);L2=parametro_robo(2); L3=parametro_robo(3);L4=parametro_robo(4);
E1=parametro_robo(5);E2=parametro_robo(6);yf=parametro_robo(8);
zf=parametro_robo(9);


q1=valor_q_inv(1);q2=valor_q_inv(2);q3=valor_q_inv(3);q4=valor_q_inv(4);
q5=valor_q_inv(5);q6=valor_q_inv(6);


 R1_0 = [cos(q1) -sin(q1) 0 0; sin(q1) cos(q1) 0 0; 0 0 1 0; 0 0 0 1];
 D1_0 = [1 0 0 E1; 0 1 0 0; 0 0 1 L1; 0 0 0 1];
 T1_0 = R1_0*D1_0;
 R2_1 = [cos(q2) 0 sin(q2) 0; 0 1 0 0; -sin(q2) 0 cos(q2) 0; 0 0 0 1];
 D2_1 = [1 0 0 L2; 0 1 0 0; 0 0 1 0; 0 0 0 1];
 T2_1 = R2_1*D2_1;
 T2_0 = T1_0*T2_1;
 R3_2 = [cos(q3) 0 sin(q3) 0; 0 1 0 0; -sin(q3) 0 cos(q3) 0; 0 0 0 1];
 D3_2 = [1 0 0 L3; 0 1 0 0; 0 0 1 E2; 0 0 0 1];
 T3_2 = R3_2*D3_2;
 T3_0 = T2_0*T3_2;
 R4_3 = [1 0 0 0; 0 cos(q4) -sin(q4) 0; 0 sin(q4) cos(q4) 0; 0 0 0 1];
 T4_3 = R4_3;
 T4_0 =T3_0*T4_3;
 R5_4 = [cos(q5) 0 sin(q5) 0; 0 1 0 0; -sin(q5) 0 cos(q5) 0; 0 0 0 1];
 T5_4 = R5_4;
 T5_0 = T4_0*T5_4;                               
 R6_5 = [1 0 0 0; 0 cos(q6) -sin(q6) 0; 0 sin(q6) cos(q6) 0; 0 0 0 1];
 T6_5 = R6_5;
 T6_0 = T5_0*T6_5; 
 D7_6 = [1 0 0 L4; 0 1 0 yf; 0 0 1 zf; 0 0 0 1];
 T7_6 = D7_6;
 T7_0=T6_0*T7_6;
 pos=T7_0(1:3,4);
posX=pos(1);
posY=pos(2);
posZ=pos(3);
end
end

== matlab function novamontagemrobo/MATLAB Function18 ==
  data: posX output; posY output; parametro_robo input; valor_q_inv input; posZ output; tarefa input; qx output; qy output; qz output; caixa input
function [posX,posY,posZ,qx,qy,qz] = pos_caixa2(parametro_robo,valor_q_inv,tarefa,caixa)
coder.extrinsic('evalin')
qx=(pi/2);
qy=(pi/2)+pi/2;
qz=0;
xf=parametro_robo(7);
posX=0;
posY=2.8-xf;
posZ=0.90764;

if caixa==2
    posX=0;
    posY=2.5-xf;
    posZ=0.90764;
end

if caixa>3
    posX=0.80015;
    posY=-2.04985+xf;
    posZ=0.24564;
    qy=0;
end

if caixa==3
qx=tarefa(4)+(pi/2);
qy=tarefa(6)+(pi/2);
qz=-tarefa(5);
L1=parametro_robo(1);L2=parametro_robo(2); L3=parametro_robo(3);L4=parametro_robo(4);
E1=parametro_robo(5);E2=parametro_robo(6);yf=parametro_robo(8);
zf=parametro_robo(9);


q1=valor_q_inv(1);q2=valor_q_inv(2);q3=valor_q_inv(3);q4=valor_q_inv(4);
q5=valor_q_inv(5);q6=valor_q_inv(6);


 R1_0 = [cos(q1) -sin(q1) 0 0; sin(q1) cos(q1) 0 0; 0 0 1 0; 0 0 0 1];
 D1_0 = [1 0 0 E1; 0 1 0 0; 0 0 1 L1; 0 0 0 1];
 T1_0 = R1_0*D1_0;
 R2_1 = [cos(q2) 0 sin(q2) 0; 0 1 0 0; -sin(q2) 0 cos(q2) 0; 0 0 0 1];
 D2_1 = [1 0 0 L2; 0 1 0 0; 0 0 1 0; 0 0 0 1];
 T2_1 = R2_1*D2_1;
 T2_0 = T1_0*T2_1;
 R3_2 = [cos(q3) 0 sin(q3) 0; 0 1 0 0; -sin(q3) 0 cos(q3) 0; 0 0 0 1];
 D3_2 = [1 0 0 L3; 0 1 0 0; 0 0 1 E2; 0 0 0 1];
 T3_2 = R3_2*D3_2;
 T3_0 = T2_0*T3_2;
 R4_3 = [1 0 0 0; 0 cos(q4) -sin(q4) 0; 0 sin(q4) cos(q4) 0; 0 0 0 1];
 T4_3 = R4_3;
 T4_0 =T3_0*T4_3;
 R5_4 = [cos(q5) 0 sin(q5) 0; 0 1 0 0; -sin(q5) 0 cos(q5) 0; 0 0 0 1];
 T5_4 = R5_4;
 T5_0 = T4_0*T5_4;                               
 R6_5 = [1 0 0 0; 0 cos(q6) -sin(q6) 0; 0 sin(q6) cos(q6) 0; 0 0 0 1];
 T6_5 = R6_5;
 T6_0 = T5_0*T6_5; 
 D7_6 = [1 0 0 L4; 0 1 0 yf; 0 0 1 zf; 0 0 0 1];
 T7_6 = D7_6;
 T7_0=T6_0*T7_6;
 pos=T7_0(1:3,4);
posX=pos(1);
posY=pos(2);
posZ=pos(3);
end
end
